simulink library "math_utils"  (R2016b)
settings: Solver=VariableStepAuto  StartTime=0.0  StopTime=10.0  RelTol=1e-3
libraries: math_utils x24, simulink x11
settings Model: Creator=jfusco1  LastModifiedBy=jfusco1

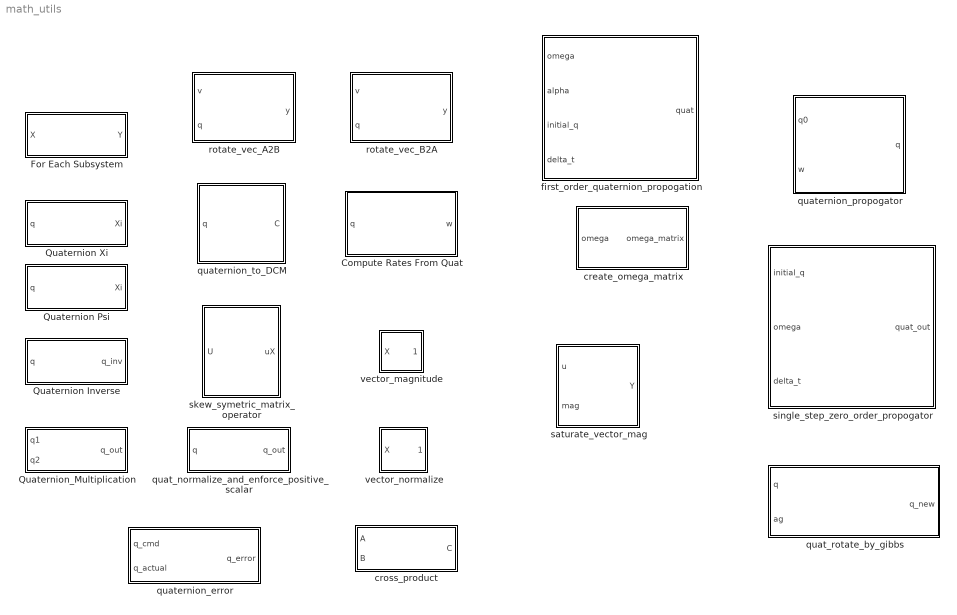
== system math_utils ==
  Compute Rates From Quat : Subsystem
      mask Display:
      | disp('Quaternion to\n\n');
      | disp('body rates');
  For Each Subsystem : Subsystem  TreatAsAtomicUnit=on  mask{T=1/62.5, omega=5, filt_enable=1}
      mask prompts: T "Sample Time:"; omega "Cutoff Freq (rad/sec):"; filt_enable "Enable Filter:"
      mask DialogControl DescTextVar Prompt: First Order Low Pass Discrete Time Filter
      mask Display: disp('1st Order Low-Pass');
  Quaternion Inverse : Subsystem
      mask Display: disp('q^{-1}', 'texmode', 'on')
  Quaternion Psi : Subsystem
      mask Display: disp('\Psi(q)', 'texmode', 'on')
  Quaternion Xi : Subsystem
      mask Display: disp('\Xi(q)', 'texmode', 'on')
  Quaternion_Multiplication : Subsystem
      mask Display: disp('q1*q2');
  create_omega_matrix : Subsystem
      mask Display: disp('\Omega(\omega)', 'tex', 'on');
  cross_product : Subsystem
      mask Display: disp('A X B = C');
  first_order_quaternion_propogation : Subsystem
      mask Display: disp('propogate(q)');
  quat_normalize_and_enforce_positive_scalar : Subsystem
      mask Display: disp('q/||q||*sign(4)')
  quat_rotate_by_gibbs : Subsystem
      mask Display: disp('rotate_quat_by_gibbs');
  quaternion_error : Subsystem
      mask Display: disp('q_{cmd} - q_{actual}', 'tex', 'on');
  quaternion_propogator : Subsystem
  quaternion_to_DCM : Subsystem
      mask Display: disp('DCM(q)');
  rotate_vec_A2B : Subsystem
      mask Display:
      | disp('Rotate Vector\n\n')
      | disp('A to B');
  rotate_vec_B2A : Subsystem
      mask Display:
      | disp('Rotate Vector\n\n')
      | disp('B to A');
  saturate_vector_mag : Subsystem
      mask Display: disp('Vector Sat');
  single_step_zero_order_propogator : Subsystem
      mask Display: disp('propogate(q,\omega)', 'tex', 'on')
  skew_symetric_matrix_operator : Subsystem
      mask Display: disp('|  u X  |');
  vector_magnitude : Subsystem
      mask Display: disp('|X|');
  vector_normalize : Subsystem
      mask Display: disp('x/||x||');

== system math_utils/Compute Rates From Quat ==
  note: Create the Xi Matrix:
      | Fundamentals of Spacecraft Attitude Determination and Control,
      | F. Landis Markley and John L. Crassidis
      | Equation: 3.21
  note: \omega = 2*\Xi^t(q)*q'
  q : Inport
  Discrete Derivative : simulink/Discrete/Discrete Derivative  gainval=1.0  ICPrevScaledInput=0.0  OutMin=[]  OutMax=[]  OutDataType=fixdt(1, 16)  OutScaling=2^-10  DoSatur=off
  Gain : Gain  Gain=2
  Math Function : Math  Operator=transpose  SaturateOnIntegerOverflow=on
  Product : Product  Multiplication=Matrix(*)
  Quaternion Xi : math_utils/Quaternion Xi  SystemSampleTime=-1
  w : Outport
  wires:
  Quaternion Xi/1 -> Math Function/1
  q/1 -> Discrete Derivative/1, Quaternion Xi/1
  Math Function/1 -> Gain/1
  Gain/1 -> Product/1
  Discrete Derivative/1 -> Product/2
  Product/1 -> w/1

== system math_utils/For Each Subsystem ==
  note: Filter derived by performing Tustin approximation of a first order Low Pass
  X : Inport  Partition=on  PartitionDimension=1  PartitionWidth=1
  3 Hz Low Pass : DiscreteTransferFcn  Numerator=[omega*T/(2+omega*T) omega*T/(2+omega*T)]  Denominator=[1 (omega*T-2)/(2+omega*T)]  SampleTime=T
  Constant : Constant  Value=filt_enable
  For Each : ForEach  DisableCoverage=on  IndexMode=One-based
  Switch : Switch  Criteria=u2 ~= 0
  Y : Outport  ConcatenationDimension=1
  wires:
  Constant/1 -> Switch/2
  3 Hz Low Pass/1 -> Switch/1
  X/1 -> Switch/3, 3 Hz Low Pass/1
  Switch/1 -> Y/1

== system math_utils/Quaternion Inverse ==
  note: Indirect Kalman Filter for 3D Attitude Estimation: A Tutorial for Aquaternion Algebra.
      | Nikolas Trawny and Stergios I. Roumeliotis
      | Equation 13
  q : Inport
  Gain : Gain  Gain=-1
  Mux : Mux  Inputs=2
  Selector : Selector  InputPortWidth=4  IndexOptions=Index vector (dialog)  Indices=[1:3]  OutputSizes=1
  Selector1 : Selector  InputPortWidth=4  IndexOptions=Index vector (dialog)  Indices=[4]  OutputSizes=1
  q_inv : Outport
  wires:
  q/1 -> Selector1/1, Selector/1
  Selector/1 -> Gain/1
  Gain/1 -> Mux/1
  Selector1/1 -> Mux/2
  Mux/1 -> q_inv/1

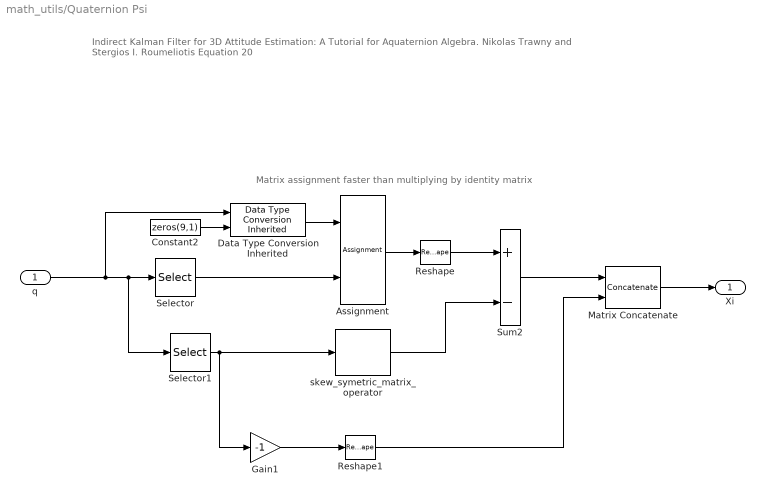
== system math_utils/Quaternion Psi ==
  note: Matrix assignment faster than multiplying by identity matrix
  note: Indirect Kalman Filter for 3D Attitude Estimation: A Tutorial for Aquaternion Algebra.
      | Nikolas Trawny and Stergios I. Roumeliotis
      | Equation 20
  q : Inport
  Assignment : Assignment  DiagnosticForDimensions=Warning  IndexOptions=Index vector (dialog)  Indices=[1 5 9]  OutputSizes=1
  Constant2 : Constant  Value=zeros(9,1)
  Data Type Conversion Inherited : simulink/Signal Attributes/Data Type Conversion Inherited  ConvertRealWorld=Real World Value  DoSatur=off
  Gain1 : Gain  Gain=-1
  Matrix Concatenate : Concatenate  Mode=Multidimensional array
  Reshape : Reshape  OutputDimensionality=Customize  OutputDimensions=[3,3]
  Reshape1 : Reshape  OutputDimensionality=Row vector (2-D)  OutputDimensions=[3,3]
  Selector : Selector  InputPortWidth=4  IndexOptions=Index vector (dialog)  Indices=[4]  OutputSizes=1
  Selector1 : Selector  InputPortWidth=4  IndexOptions=Index vector (dialog)  Indices=[1:3]  OutputSizes=1
  Sum2 : Sum  Inputs=+-
  skew_symetric_matrix_operator : math_utils/skew_symetric_matrix_operator  SystemSampleTime=-1
  Xi : Outport
  wires:
  Selector/1 -> Assignment/2
  Assignment/1 -> Reshape/1
  Reshape/1 -> Sum2/1
  q/1 -> Data Type Conversion Inherited/1, Selector1/1, Selector/1
  Selector1/1 -> skew_symetric_matrix_operator/1, Gain1/1
  skew_symetric_matrix_operator/1 -> Sum2/2
  Gain1/1 -> Reshape1/1
  Sum2/1 -> Matrix Concatenate/1
  Reshape1/1 -> Matrix Concatenate/2
  Matrix Concatenate/1 -> Xi/1
  Constant2/1 -> Data Type Conversion Inherited/2
  Data Type Conversion Inherited/1 -> Assignment/1

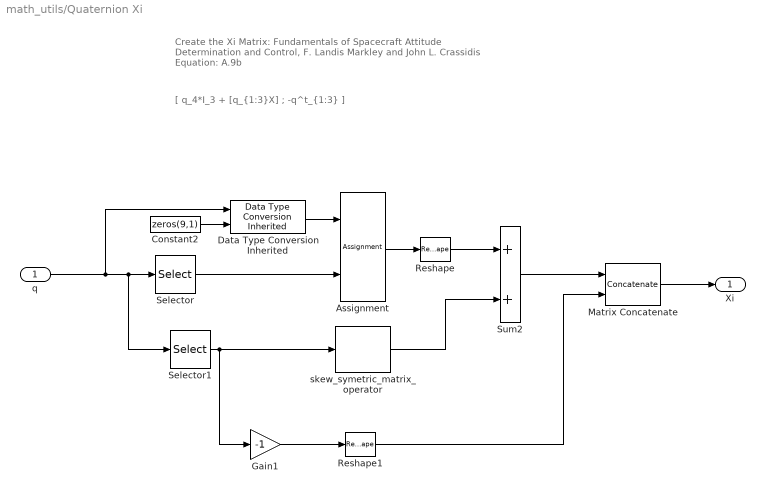
== system math_utils/Quaternion Xi ==
  note: Create the Xi Matrix:
      | Fundamentals of Spacecraft Attitude Determination and Control,
      | F. Landis Markley and John L. Crassidis
      | Equation: A.9b
  note: [ q_4*I_3 + [q_{1:3}X] ;
      |  -q^t_{1:3} ]
  q : Inport
  Assignment : Assignment  DiagnosticForDimensions=Warning  IndexOptions=Index vector (dialog)  Indices=[1 5 9]  OutputSizes=1
  Constant2 : Constant  Value=zeros(9,1)
  Data Type Conversion Inherited : simulink/Signal Attributes/Data Type Conversion Inherited  ConvertRealWorld=Real World Value  DoSatur=off
  Gain1 : Gain  Gain=-1
  Matrix Concatenate : Concatenate  Mode=Multidimensional array
  Reshape : Reshape  OutputDimensionality=Customize  OutputDimensions=[3,3]
  Reshape1 : Reshape  OutputDimensionality=Row vector (2-D)  OutputDimensions=[3,3]
  Selector : Selector  InputPortWidth=4  IndexOptions=Index vector (dialog)  Indices=[4]  OutputSizes=1
  Selector1 : Selector  InputPortWidth=4  IndexOptions=Index vector (dialog)  Indices=[1:3]  OutputSizes=1
  Sum2 : Sum
  skew_symetric_matrix_operator : math_utils/skew_symetric_matrix_operator  SystemSampleTime=-1
  Xi : Outport
  wires:
  Selector/1 -> Assignment/2
  Assignment/1 -> Reshape/1
  Reshape/1 -> Sum2/1
  q/1 -> Data Type Conversion Inherited/1, Selector1/1, Selector/1
  Selector1/1 -> skew_symetric_matrix_operator/1, Gain1/1
  skew_symetric_matrix_operator/1 -> Sum2/2
  Gain1/1 -> Reshape1/1
  Sum2/1 -> Matrix Concatenate/1
  Reshape1/1 -> Matrix Concatenate/2
  Matrix Concatenate/1 -> Xi/1
  Constant2/1 -> Data Type Conversion Inherited/2
  Data Type Conversion Inherited/1 -> Assignment/1

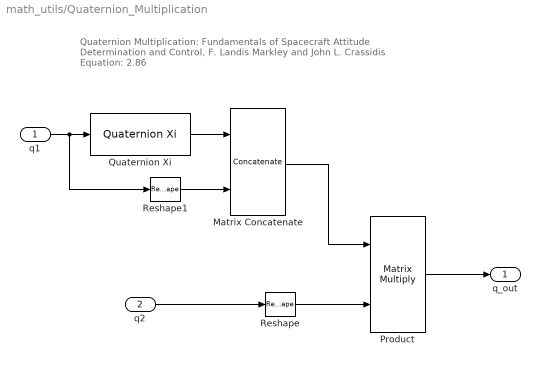
== system math_utils/Quaternion_Multiplication ==
  note: Quaternion Multiplication:
      | Fundamentals of Spacecraft Attitude Determination and Control,
      | F. Landis Markley and John L. Crassidis
      | Equation: 2.86
  q1 : Inport
  q2 : Inport  Port=2
  Matrix Concatenate : Concatenate  Mode=Multidimensional array  ConcatenateDimension=2
  Product : Product  Multiplication=Matrix(*)
  Quaternion Xi : math_utils/Quaternion Xi  SystemSampleTime=-1
  Reshape : Reshape  OutputDimensionality=Column vector (2-D)
  Reshape1 : Reshape  OutputDimensionality=Column vector (2-D)
  q_out : Outport
  wires:
  q1/1 -> Reshape1/1, Quaternion Xi/1
  Reshape/1 -> Product/2
  q2/1 -> Reshape/1
  Quaternion Xi/1 -> Matrix Concatenate/1
  Reshape1/1 -> Matrix Concatenate/2
  Matrix Concatenate/1 -> Product/1
  Product/1 -> q_out/1

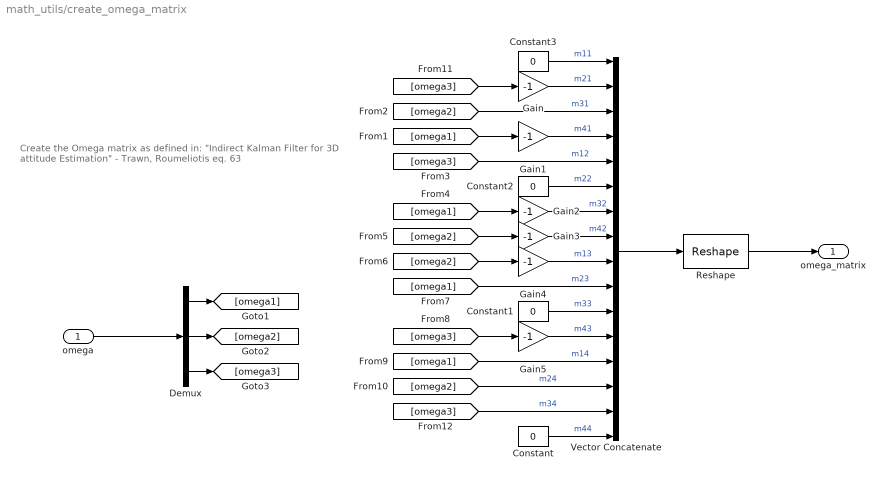
== system math_utils/create_omega_matrix ==
  note: Create the Omega matrix as defined in:
      | "Indirect Kalman Filter for 3D attitude Estimation" - Trawn, Roumeliotis
      | eq. 63
  omega : Inport  PortDimensions=3
  Constant{,1..3} (4 alike) : Constant  Value=0  OutDataTypeStr=Inherit: Inherit via back propagation
  Demux : Demux  Outputs=3
  Gain{,1..5} (6 alike) : Gain  Gain=-1
  Reshape : Reshape  OutputDimensionality=Customize  OutputDimensions=[4,4]
  Vector Concatenate : Concatenate  NumInputs=16
  omega_matrix : Outport
  wires:
  [omega3] -> Gain5/1
  [omega2] -> Gain4/1
  [omega1] -> Gain2/1
  [omega2] -> Gain3/1
  [omega1] -> Gain1/1
  [omega3] -> Gain/1
  Reshape/1 -> omega_matrix/1
  [omega3] -> Vector Concatenate/15  "m34"
  [omega2] -> Vector Concatenate/14  "m24"
  [omega1] -> Vector Concatenate/13  "m14"
  Gain5/1 -> Vector Concatenate/12  "m43"
  Constant/1 -> Vector Concatenate/16  "m44"
  Constant1/1 -> Vector Concatenate/11  "m33"
  [omega1] -> Vector Concatenate/10  "m23"
  Gain4/1 -> Vector Concatenate/9  "m13"
  Gain3/1 -> Vector Concatenate/8  "m42"
  Gain2/1 -> Vector Concatenate/7  "m32"
  [omega3] -> Vector Concatenate/5  "m12"
  [omega2] -> Vector Concatenate/3  "m31"
  Gain1/1 -> Vector Concatenate/4  "m41"
  Constant2/1 -> Vector Concatenate/6  "m22"
  Gain/1 -> Vector Concatenate/2  "m21"
  Constant3/1 -> Vector Concatenate/1  "m11"
  Vector Concatenate/1 -> Reshape/1
  Demux/3 -> [omega3]
  Demux/2 -> [omega2]
  Demux/1 -> [omega1]
  omega/1 -> Demux/1

== system math_utils/cross_product ==
  A : Inport
  B : Inport  Port=2
  Product : Product  Multiplication=Matrix(*)
  skew_symetric_matrix_operator : math_utils/skew_symetric_matrix_operator  SystemSampleTime=-1
  C : Outport
  wires:
  A/1 -> skew_symetric_matrix_operator/1
  skew_symetric_matrix_operator/1 -> Product/1
  B/1 -> Product/2
  Product/1 -> C/1

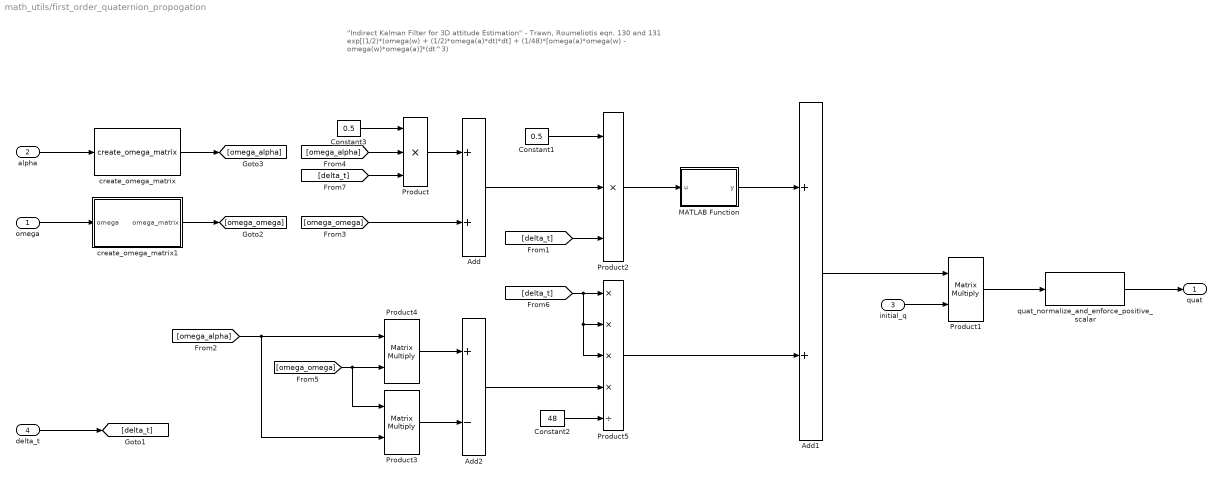
== system math_utils/first_order_quaternion_propogation ==
  note: "Indirect Kalman Filter for 3D attitude Estimation" - Trawn, Roumeliotis
      | eqn. 130 and 131
      |
      | exp[(1/2)*(omega(w) + (1/2)*omega(a)*dt)*dt] + (1/48)*[omega(a)*omega(w) - omega(w)*omega(a)]*(dt^3)
  omega : Inport  PortDimensions=3
  alpha : Inport  Port=2  PortDimensions=3
  initial_q : Inport  Port=3  OutMin=-[1]  OutMax=[1]  PortDimensions=4
  delta_t : Inport  Port=4  PortDimensions=1
  Add : Sum
  Add1 : Sum
  Add2 : Sum  Inputs=+-
  Constant1 : Constant  Value=0.5  OutDataTypeStr=Inherit: Inherit via back propagation
  Constant2 : Constant  Value=48  OutDataTypeStr=Inherit: Inherit via back propagation
  Constant3 : Constant  Value=0.5  OutDataTypeStr=Inherit: Inherit via back propagation
  MATLAB Function : MATLAB Function  TreatAsAtomicUnit=on
  Product : Product  Inputs=3
  Product1 : Product  Multiplication=Matrix(*)  RndMeth=Zero
  Product2 : Product  Inputs=3
  Product3 : Product  Multiplication=Matrix(*)  RndMeth=Zero
  Product4 : Product  Multiplication=Matrix(*)  RndMeth=Zero
  Product5 : Product  Inputs=****/
  create_omega_matrix : math_utils/create_omega_matrix  SystemSampleTime=-1
  create_omega_matrix1 : Subsystem
      mask Display: disp('\Omega(\omega)', 'tex', 'on');
  quat_normalize_and_enforce_positive_scalar : math_utils/quat_normalize_and_enforce_positive_scalar  SystemSampleTime=-1
  quat : Outport  OutMin=-[1]  OutMax=[1]  PortDimensions=4
  wires:
  Product5/1 -> Add1/2
  [delta_t] -> Product5/3, Product5/2, Product5/1
  Constant2/1 -> Product5/5
  Add2/1 -> Product5/4
  [omega_omega] -> Product4/2, Product3/1
  Product3/1 -> Add2/2
  Product4/1 -> Add2/1
  [omega_alpha] -> Product4/1, Product3/2
  create_omega_matrix/1 -> [omega_alpha]
  [omega_alpha] -> Product/2
  [omega_omega] -> Add/2
  create_omega_matrix1/1(omega_matrix) -> [omega_omega]
  MATLAB Function/1(y) -> Add1/1
  Product2/1 -> MATLAB Function/1(u)
  [delta_t] -> Product2/3
  Add/1 -> Product2/2
  Constant1/1 -> Product2/1
  Product/1 -> Add/1
  [delta_t] -> Product/3
  delta_t/1 -> [delta_t]
  Constant3/1 -> Product/1
  alpha/1 -> create_omega_matrix/1
  omega/1 -> create_omega_matrix1/1(omega)
  initial_q/1 -> Product1/2
  Add1/1 -> Product1/1
  Product1/1 -> quat_normalize_and_enforce_positive_scalar/1
  quat_normalize_and_enforce_positive_scalar/1 -> quat/1

== system math_utils/quat_normalize_and_enforce_positive_scalar ==
  note: It is sometimes desirable to enforce that the scalar component of a quaternion is positive.
      | The scalar dithering between positive and negative can lead to numerical issues with
      | some quaternion operations.
  q : Inport  PortDimensions=4
  If : If  IfExpression=u1 < 0
  Merge : Merge
  No-op : Subsystem  TreatAsAtomicUnit=on
  Normalize : Subsystem  TreatAsAtomicUnit=on
  Selector : Selector  InputPortWidth=4  IndexOptions=Index vector (dialog)  Indices=[4]  OutputSizes=1
  vector_normalize : math_utils/vector_normalize  SystemSampleTime=-1
  q_out : Outport
  wires:
  q/1 -> No-op/1(In1), Normalize/1(q_in), Selector/1
  Selector/1 -> If/1
  If/2 -> No-op/Action
  If/1 -> Normalize/Action
  Normalize/1(positive_scalar_q) -> Merge/1
  No-op/1(Out1) -> Merge/2
  Merge/1 -> vector_normalize/1
  vector_normalize/1 -> q_out/1

== system math_utils/quat_rotate_by_gibbs ==
  note: q _{filt} = [ a_g ; 2 ]
  note: q _{sc} = q_{ref} \otimes q_{filt}
  note: Convert gibbs vector to quaternion attitue using the reference quaternion
  note: Rotate a quaternion by a gibbs vector.
      |
      | Attitude Error Representations for Kalman Filtering
      | F. Landis Markley
      | Equation: 21
  q : Inport  PortDimensions=4
  ag : Inport  Port=2  PortDimensions=3
  Constant1 : Constant  Value=single(2)
  Quaternion_Multiplication : math_utils/Quaternion_Multiplication  SystemSampleTime=-1
  Vector Concatenate : Concatenate
  quat_normalize_and_enforce_positive_scalar : math_utils/quat_normalize_and_enforce_positive_scalar  SystemSampleTime=-1
  q_new : Outport  PortDimensions=4
  wires:
  Constant1/1 -> Vector Concatenate/2
  Vector Concatenate/1 -> Quaternion_Multiplication/2
  Quaternion_Multiplication/1 -> quat_normalize_and_enforce_positive_scalar/1
  q/1 -> Quaternion_Multiplication/1
  ag/1 -> Vector Concatenate/1
  quat_normalize_and_enforce_positive_scalar/1 -> q_new/1

== system math_utils/quaternion_error ==
  note: Calculate Quaternion Error For Feedback Control:
      | Fundamentals of Spacecraft Attitude Determination and Control,
      | F. Landis Markley and John L. Crassidis
      | Equation: 7.4 and 7.13 combined. Eq 7.4 was modified to use Hamilton's quaternion multiplicatoin convention.
  q_cmd : Inport
  q_actual : Inport  Port=2
  Quaternion Inverse : math_utils/Quaternion Inverse  SystemSampleTime=-1
  Quaternion_Multiplication : math_utils/Quaternion_Multiplication  SystemSampleTime=-1
  quat_normalize_and_enforce_positive_scalar : math_utils/quat_normalize_and_enforce_positive_scalar  SystemSampleTime=-1
  q_error : Outport
  wires:
  q_actual/1 -> Quaternion Inverse/1
  Quaternion Inverse/1 -> Quaternion_Multiplication/1
  q_cmd/1 -> Quaternion_Multiplication/2
  quat_normalize_and_enforce_positive_scalar/1 -> q_error/1
  Quaternion_Multiplication/1 -> quat_normalize_and_enforce_positive_scalar/1

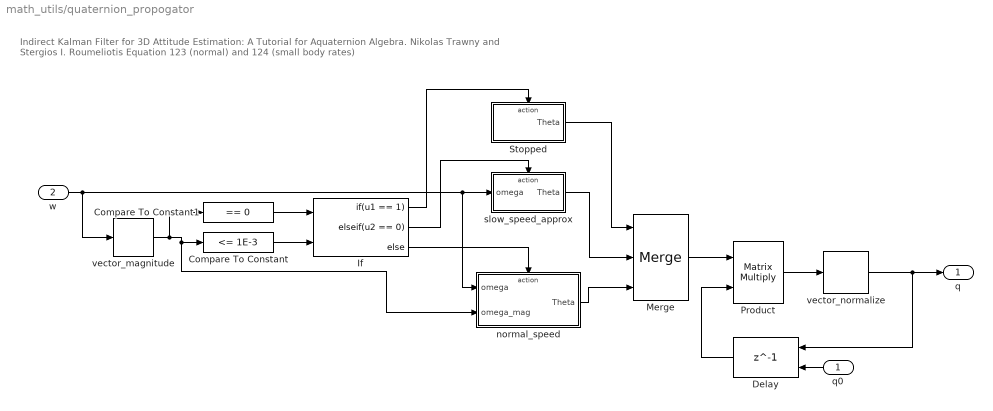
== system math_utils/quaternion_propogator ==
  note: Indirect Kalman Filter for 3D Attitude Estimation: A Tutorial for Aquaternion Algebra.
      | Nikolas Trawny and Stergios I. Roumeliotis
      | Equation 123 (normal) and 124 (small body rates)
  q0 : Inport
  w : Inport  Port=2
  Compare To Constant : simulink/Logic and Bit Operations/Compare To Constant  relop=<=  const=1E-3  OutDataTypeStr=boolean
  Compare To Constant1 : simulink/Logic and Bit Operations/Compare To Constant  relop===  const=0  OutDataTypeStr=boolean
  Delay : Delay  DelayLength=1  InitialConditionSource=Input port
      settings: InputPortMap=u0,p4
  If : If  NumInputs=2  IfExpression=u1 == 1  ElseIfExpressions=u2 == 0
  Merge : Merge  Inputs=3
  Product : Product  Multiplication=Matrix(*)
  Stopped : Subsystem  TreatAsAtomicUnit=on
  normal_speed : Subsystem  TreatAsAtomicUnit=on
  slow_speed_approx : Subsystem  TreatAsAtomicUnit=on
  vector_magnitude : math_utils/vector_magnitude  SystemSampleTime=-1
  vector_normalize : math_utils/vector_normalize  SystemSampleTime=-1
  q : Outport
  wires:
  w/1 -> vector_magnitude/1, normal_speed/1("omega "), slow_speed_approx/1(omega)
  q0/1 -> Delay/2
  Compare To Constant/1 -> If/2
  vector_magnitude/1 -> Compare To Constant1/1, normal_speed/2(omega_mag), Compare To Constant/1
  If/2 -> slow_speed_approx/Action
  If/3 -> normal_speed/Action
  slow_speed_approx/1(Theta) -> Merge/2
  normal_speed/1(Theta) -> Merge/3
  Merge/1 -> Product/1
  Product/1 -> vector_normalize/1
  vector_normalize/1 -> q/1, Delay/1
  Delay/1 -> Product/2
  Compare To Constant1/1 -> If/1
  If/1 -> Stopped/Action
  Stopped/1(Theta) -> Merge/1

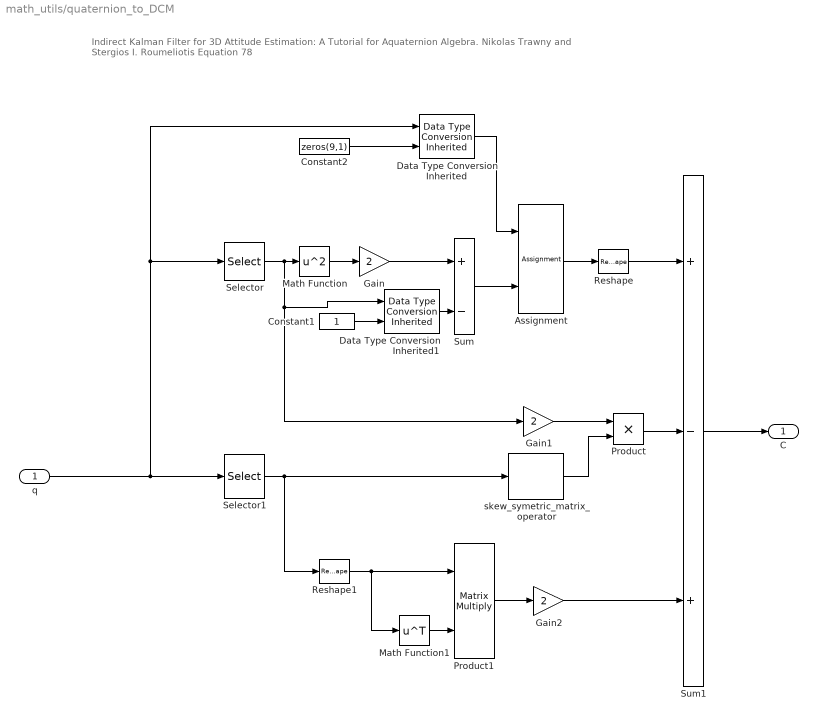
== system math_utils/quaternion_to_DCM ==
  note: Indirect Kalman Filter for 3D Attitude Estimation: A Tutorial for Aquaternion Algebra.
      | Nikolas Trawny and Stergios I. Roumeliotis
      | Equation 78
  q : Inport  PortDimensions=4
  Assignment : Assignment  DiagnosticForDimensions=Warning  IndexOptions=Index vector (dialog)  Indices=[1 5 9]  OutputSizes=1
  Constant1 : Constant
  Constant2 : Constant  Value=zeros(9,1)
  Data Type Conversion Inherited : simulink/Signal Attributes/Data Type Conversion Inherited  ConvertRealWorld=Real World Value  DoSatur=off
  Data Type Conversion Inherited1 : simulink/Signal Attributes/Data Type Conversion Inherited  ConvertRealWorld=Real World Value  DoSatur=off
  Gain : Gain  Gain=2
  Gain1 : Gain  Gain=2
  Gain2 : Gain  Gain=2
  Math Function : Math  Operator=square  SaturateOnIntegerOverflow=on
  Math Function1 : Math  Operator=transpose  SaturateOnIntegerOverflow=on
  Product : Product
  Product1 : Product  Multiplication=Matrix(*)
  Reshape : Reshape  OutputDimensionality=Customize  OutputDimensions=[3,3]
  Reshape1 : Reshape  OutputDimensionality=Column vector (2-D)  OutputDimensions=[3,3]
  Selector : Selector  InputPortWidth=4  IndexOptions=Index vector (dialog)  Indices=[4]  OutputSizes=1
  Selector1 : Selector  InputPortWidth=4  IndexOptions=Index vector (dialog)  Indices=[1 2 3]  OutputSizes=1
  Sum : Sum  Inputs=+-
  Sum1 : Sum  Inputs=+-+
  skew_symetric_matrix_operator : math_utils/skew_symetric_matrix_operator  SystemSampleTime=-1
  C : Outport
  wires:
  Selector/1 -> Data Type Conversion Inherited1/1, Gain1/1, Math Function/1
  Sum/1 -> Assignment/2
  Math Function/1 -> Gain/1
  Assignment/1 -> Reshape/1
  Gain/1 -> Sum/1
  Reshape/1 -> Sum1/1
  Selector1/1 -> Reshape1/1, skew_symetric_matrix_operator/1
  Gain1/1 -> Product/1
  skew_symetric_matrix_operator/1 -> Product/2
  Product/1 -> Sum1/2
  Math Function1/1 -> Product1/2
  q/1 -> Selector1/1, Selector/1, Data Type Conversion Inherited/1
  Product1/1 -> Gain2/1
  Gain2/1 -> Sum1/3
  Sum1/1 -> C/1
  Reshape1/1 -> Math Function1/1, Product1/1
  Constant2/1 -> Data Type Conversion Inherited/2
  Data Type Conversion Inherited/1 -> Assignment/1
  Data Type Conversion Inherited1/1 -> Sum/2
  Constant1/1 -> Data Type Conversion Inherited1/2

== system math_utils/rotate_vec_A2B ==
  note: Rotate a vector from Frame A to Frame B using a rotation matrix.
  v : Inport
  q : Inport  Port=2  PortDimensions=4
  Product : Product  Multiplication=Matrix(*)
  quaternion_to_DCM : math_utils/quaternion_to_DCM  SystemSampleTime=-1
  y : Outport
  wires:
  q/1 -> quaternion_to_DCM/1
  quaternion_to_DCM/1 -> Product/1
  v/1 -> Product/2
  Product/1 -> y/1

== system math_utils/rotate_vec_B2A ==
  note: Rotate a vector from Frame B to Frame A using the tranpose of a rotation matrix.
  v : Inport
  q : Inport  Port=2
  Math Function : Math  Operator=transpose  SaturateOnIntegerOverflow=on
  Product : Product  Multiplication=Matrix(*)
  quaternion_to_DCM : math_utils/quaternion_to_DCM  SystemSampleTime=-1
  y : Outport
  wires:
  Product/1 -> y/1
  v/1 -> Product/2
  quaternion_to_DCM/1 -> Math Function/1
  q/1 -> quaternion_to_DCM/1
  Math Function/1 -> Product/1

== system math_utils/saturate_vector_mag ==
  note: This block saturates the vector (u) magnitude at the value specified by 'mag'
      | If the magnitude of U is less than the threshold, the vector is passed.
      | If the vector has a greater magnitude than the threshold then the magnitude of the vector is reduced to that threshold magnitude
  u : Inport
  mag : Inport  Port=2
  Product : Product
  Relational Operator : RelationalOperator  Operator=<  OutDataTypeStr=boolean  RndMeth=Nearest
  Switch : Switch  Criteria=u2 ~= 0
  vector_magnitude1 : math_utils/vector_magnitude  SystemSampleTime=-1
  vector_normalize : math_utils/vector_normalize  SystemSampleTime=-1
  Y : Outport
  wires:
  u/1 -> Switch/1, vector_normalize/1, vector_magnitude1/1
  mag/1 -> Product/1, Relational Operator/2
  vector_magnitude1/1 -> Relational Operator/1
  Relational Operator/1 -> Switch/2
  Product/1 -> Switch/3
  Switch/1 -> Y/1
  vector_normalize/1 -> Product/2

== system math_utils/single_step_zero_order_propogator ==
  initial_q : Inport
  omega : Inport  Port=2
  delta_t : Inport  Port=3
  Constant : Constant  Value=[0 0 0]
  Data Type Conversion Inherited : simulink/Signal Attributes/Data Type Conversion Inherited  ConvertRealWorld=Real World Value  DoSatur=off
  first_order_quaternion_propogation : math_utils/first_order_quaternion_propogation  SystemSampleTime=-1
  quat_out : Outport
  wires:
  first_order_quaternion_propogation/1 -> quat_out/1
  Constant/1 -> Data Type Conversion Inherited/2
  initial_q/1 -> first_order_quaternion_propogation/3, Data Type Conversion Inherited/1
  omega/1 -> first_order_quaternion_propogation/1
  delta_t/1 -> first_order_quaternion_propogation/4
  Data Type Conversion Inherited/1 -> first_order_quaternion_propogation/2

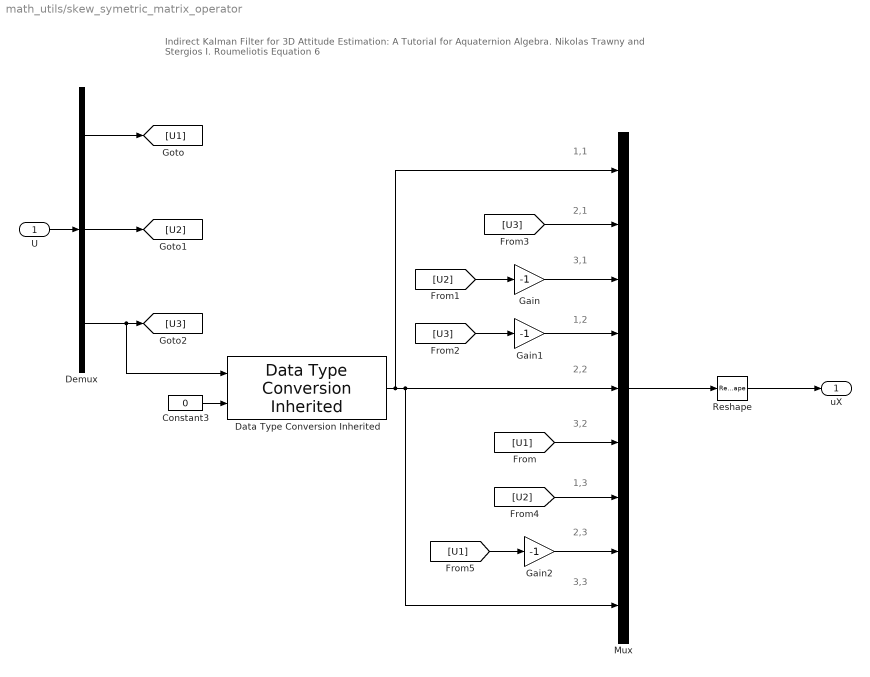
== system math_utils/skew_symetric_matrix_operator ==
  note: 1,1
  note: Indirect Kalman Filter for 3D Attitude Estimation: A Tutorial for Aquaternion Algebra.
      | Nikolas Trawny and Stergios I. Roumeliotis
      | Equation 6
  note: 2,1
  note: 3,1
  note: 1,2
  note: 2,2
  note: 3,2
  note: 1,3
  note: 2,3
  note: 3,3
  U : Inport  PortDimensions=3
  Constant3 : Constant  Value=0
  Data Type Conversion Inherited : simulink/Signal Attributes/Data Type Conversion Inherited  ConvertRealWorld=Real World Value  DoSatur=off
  Demux : Demux  Outputs=3
  Gain : Gain  Gain=-1
  Gain1 : Gain  Gain=-1
  Gain2 : Gain  Gain=-1
  Mux : Mux  Inputs=9
  Reshape : Reshape  OutputDimensionality=Customize  OutputDimensions=[3,3]
  uX : Outport
  wires:
  U/1 -> Demux/1
  Demux/1 -> [U1]
  Demux/2 -> [U2]
  Demux/3 -> Data Type Conversion Inherited/1, [U3]
  [U3] -> Mux/2
  [U2] -> Gain/1
  Gain/1 -> Mux/3
  Gain1/1 -> Mux/4
  [U3] -> Gain1/1
  [U1] -> Mux/6
  [U2] -> Mux/7
  Gain2/1 -> Mux/8
  [U1] -> Gain2/1
  Data Type Conversion Inherited/1 -> Mux/1, Mux/9, Mux/5
  Mux/1 -> Reshape/1
  Constant3/1 -> Data Type Conversion Inherited/2
  Reshape/1 -> uX/1

== system math_utils/vector_magnitude ==
  note: Compute the magnitude of a vector
  X : Inport
  Dot Product : DotProduct  InputSameDT=on  OutDataTypeStr=Inherit: Inherit via internal rule
  Sqrt : Sqrt  SaturateOnIntegerOverflow=on
  X_out : Outport
  wires:
  X/1 -> Dot Product/1, Dot Product/2
  Dot Product/1 -> Sqrt/1
  Sqrt/1 -> X_out/1

== system math_utils/vector_normalize ==
  note: Protect against dividing by zero.
      | If the vector magnitude is below a threshold just pass the vector
  X : Inport
  Data Type Conversion : DataTypeConversion  OutDataTypeStr=double
  If : If  IfExpression=u1 > 1E-7
  Merge : Merge
  No-op : Subsystem  TreatAsAtomicUnit=on
  Normalize : Subsystem  TreatAsAtomicUnit=on
  vector_magnitude : math_utils/vector_magnitude  SystemSampleTime=-1
  X_norm : Outport
  wires:
  X/1 -> No-op/1(In1), vector_magnitude/1, Normalize/1(Vec)
  vector_magnitude/1 -> Data Type Conversion/1, Normalize/2(Magnitude)
  If/2 -> No-op/Action
  If/1 -> Normalize/Action
  Normalize/1(Normalized_Vec) -> Merge/1
  No-op/1(Out1) -> Merge/2
  Merge/1 -> X_norm/1
  Data Type Conversion/1 -> If/1

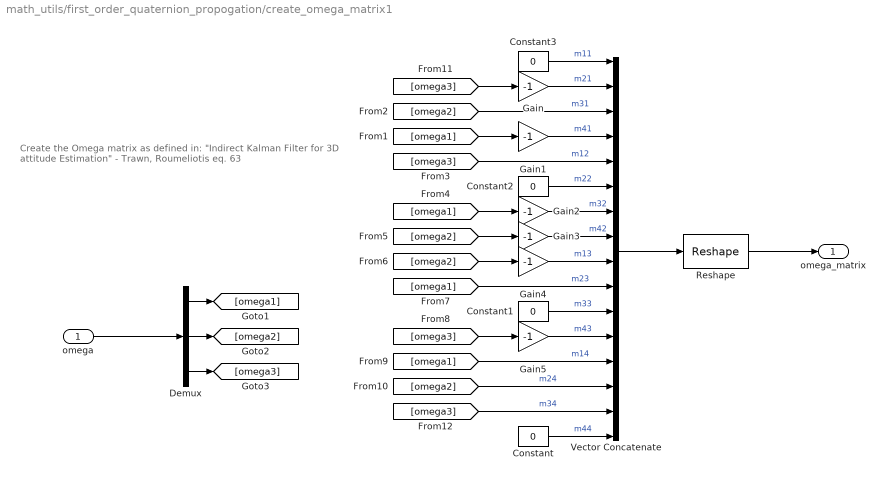
== system math_utils/first_order_quaternion_propogation/create_omega_matrix1 ==
  note: Create the Omega matrix as defined in:
      | "Indirect Kalman Filter for 3D attitude Estimation" - Trawn, Roumeliotis
      | eq. 63
  omega : Inport  PortDimensions=3
  Constant{,1..3} (4 alike) : Constant  Value=0  OutDataTypeStr=Inherit: Inherit via back propagation
  Demux : Demux  Outputs=3
  Gain{,1..5} (6 alike) : Gain  Gain=-1
  Reshape : Reshape  OutputDimensionality=Customize  OutputDimensions=[4,4]
  Vector Concatenate : Concatenate  NumInputs=16
  omega_matrix : Outport
  wires:
  omega/1 -> Demux/1
  Demux/1 -> [omega1]
  Demux/2 -> [omega2]
  Demux/3 -> [omega3]
  Vector Concatenate/1 -> Reshape/1
  Constant3/1 -> Vector Concatenate/1  "m11"
  Gain/1 -> Vector Concatenate/2  "m21"
  Constant2/1 -> Vector Concatenate/6  "m22"
  Gain1/1 -> Vector Concatenate/4  "m41"
  [omega2] -> Vector Concatenate/3  "m31"
  [omega3] -> Vector Concatenate/5  "m12"
  Gain2/1 -> Vector Concatenate/7  "m32"
  Gain3/1 -> Vector Concatenate/8  "m42"
  Gain4/1 -> Vector Concatenate/9  "m13"
  [omega1] -> Vector Concatenate/10  "m23"
  Constant1/1 -> Vector Concatenate/11  "m33"
  Constant/1 -> Vector Concatenate/16  "m44"
  Gain5/1 -> Vector Concatenate/12  "m43"
  [omega1] -> Vector Concatenate/13  "m14"
  [omega2] -> Vector Concatenate/14  "m24"
  [omega3] -> Vector Concatenate/15  "m34"
  Reshape/1 -> omega_matrix/1
  [omega3] -> Gain/1
  [omega1] -> Gain1/1
  [omega2] -> Gain3/1
  [omega1] -> Gain2/1
  [omega2] -> Gain4/1
  [omega3] -> Gain5/1

== system math_utils/quat_normalize_and_enforce_positive_scalar/No-op ==
  In1 : Inport
  Action Port : ActionPort  ActionType=else
  Out1 : Outport
  wires:
  In1/1 -> Out1/1

== system math_utils/quat_normalize_and_enforce_positive_scalar/Normalize ==
  q_in : Inport
  Action Port : ActionPort  ActionType=then
  Constant1 : Constant  Value=-1
  Data Type Conversion Inherited : simulink/Signal Attributes/Data Type Conversion Inherited  ConvertRealWorld=Real World Value  DoSatur=off
  Product : Product
  positive_scalar_q : Outport
  wires:
  q_in/1 -> Product/1, Data Type Conversion Inherited/1
  Constant1/1 -> Data Type Conversion Inherited/2
  Data Type Conversion Inherited/1 -> Product/2
  Product/1 -> positive_scalar_q/1

== system math_utils/quaternion_propogator/Stopped ==
  Action Port : ActionPort  ActionType=then
  Constant : Constant  Value=eye(4)  OutDataTypeStr=Inherit: Inherit via back propagation
  Theta : Outport
  wires:
  Constant/1 -> Theta/1

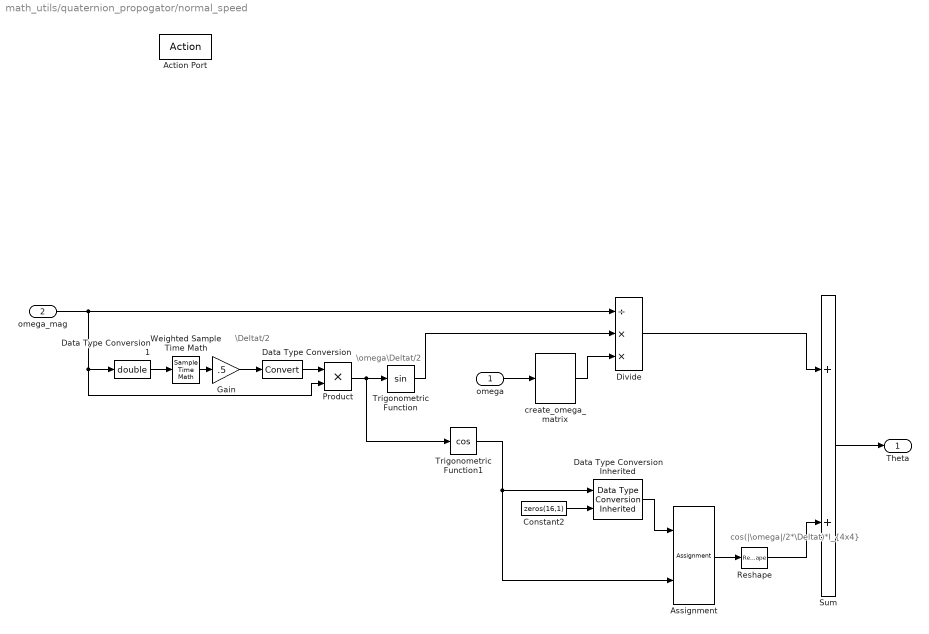
== system math_utils/quaternion_propogator/normal_speed ==
  note: cos(|\omega|/2*\Deltat)*I_{4x4}
  note: \Deltat/2
  note: \omega\Deltat/2
  "omega " : Inport
  omega_mag : Inport  Port=2
  Action Port : ActionPort  ActionType=else
  Assignment : Assignment  DiagnosticForDimensions=Warning  IndexOptions=Index vector (dialog)  Indices=[1 6 11 16]  OutputSizes=1
  Constant2 : Constant  Value=zeros(16,1)
  Data Type Conversion Inherited : simulink/Signal Attributes/Data Type Conversion Inherited  ConvertRealWorld=Real World Value  DoSatur=off
  Data Type Conversion : DataTypeConversion
  Data Type Conversion1 : DataTypeConversion  OutDataTypeStr=double
  Divide : Product  Inputs=/**
  Gain : Gain  Gain=.5
  Product : Product
  Reshape : Reshape  OutputDimensionality=Customize  OutputDimensions=[4,4]
  Sum : Sum
  Trigonometric Function : Trigonometry
  Trigonometric Function1 : Trigonometry  Operator=cos
  Weighted Sample Time Math : SampleTimeMath  TsampMathOp=Ts Only
  create_omega_matrix : math_utils/create_omega_matrix  SystemSampleTime=-1
  Theta : Outport
  wires:
  omega_mag/1 -> Product/2, Data Type Conversion1/1, Divide/1
  Data Type Conversion1/1 -> Weighted Sample Time Math/1
  Weighted Sample Time Math/1 -> Gain/1
  Gain/1 -> Data Type Conversion/1
  Data Type Conversion/1 -> Product/1
  Trigonometric Function/1 -> Divide/2
  Product/1 -> Trigonometric Function1/1, Trigonometric Function/1
  Trigonometric Function1/1 -> Assignment/2, Data Type Conversion Inherited/1
  Constant2/1 -> Data Type Conversion Inherited/2
  Data Type Conversion Inherited/1 -> Assignment/1
  Assignment/1 -> Reshape/1
  "omega "/1 -> create_omega_matrix/1
  create_omega_matrix/1 -> Divide/3
  Reshape/1 -> Sum/2
  Divide/1 -> Sum/1
  Sum/1 -> Theta/1

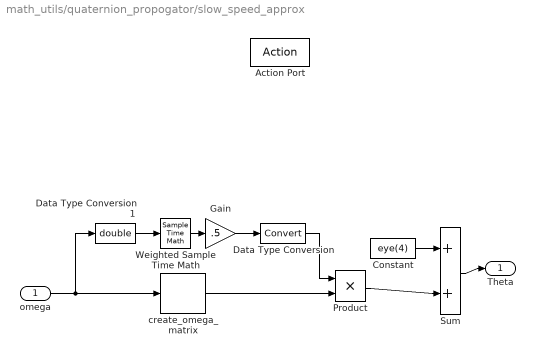
== system math_utils/quaternion_propogator/slow_speed_approx ==
  omega : Inport
  Action Port : ActionPort  ActionType=elseif
  Constant : Constant  Value=eye(4)  OutDataTypeStr=Inherit: Inherit via back propagation
  Data Type Conversion : DataTypeConversion
  Data Type Conversion1 : DataTypeConversion  OutDataTypeStr=double
  Gain : Gain  Gain=.5
  Product : Product
  Sum : Sum
  Weighted Sample Time Math : SampleTimeMath  TsampMathOp=Ts Only
  create_omega_matrix : math_utils/create_omega_matrix  SystemSampleTime=-1
  Theta : Outport
  wires:
  Constant/1 -> Sum/1
  omega/1 -> Data Type Conversion1/1, create_omega_matrix/1
  Data Type Conversion1/1 -> Weighted Sample Time Math/1
  Weighted Sample Time Math/1 -> Gain/1
  Gain/1 -> Data Type Conversion/1
  Product/1 -> Sum/2
  Data Type Conversion/1 -> Product/1
  create_omega_matrix/1 -> Product/2
  Sum/1 -> Theta/1

== system math_utils/vector_normalize/No-op ==
  In1 : Inport
  Action Port : ActionPort  ActionType=else
  Out1 : Outport
  wires:
  In1/1 -> Out1/1

== system math_utils/vector_normalize/Normalize ==
  Vec : Inport
  Magnitude : Inport  Port=2
  Action Port : ActionPort  ActionType=then
  Divide : Product  Inputs=*/
  Normalized_Vec : Outport
  wires:
  Vec/1 -> Divide/1
  Magnitude/1 -> Divide/2
  Divide/1 -> Normalized_Vec/1

== matlab function math_utils/first_order_quaternion_propogation/MATLAB Function ==
  data: u input; y output
function y = expm(u)
%#codegen

y = expm(u);
